simulink model "E_ZH_Z5"  (R2025a)
settings: Solver=VariableStepAuto  StartTime=0.0  StopTime=10.0  RelTol=1e-3
libraries: simulink x2, ZH_Z x1
settings Model: Creator=Szalay  LastModifiedBy=Szalay
settings RTWCC: RTWVerbose=off

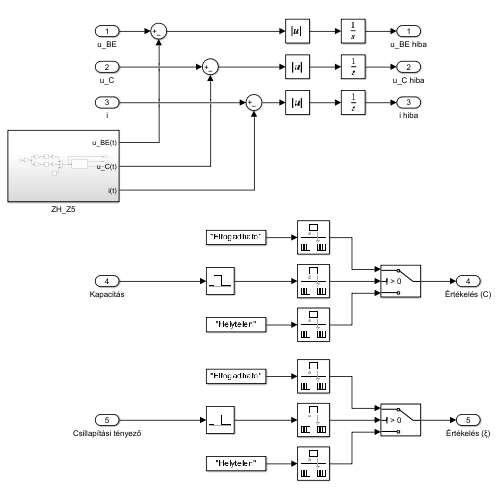
[thumbnail: Simulink's stored preview of the top-level diagram]
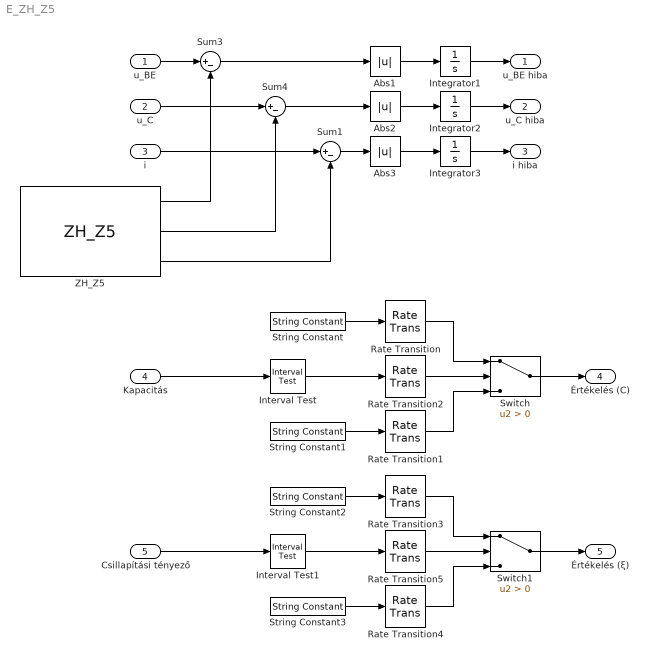
== system E_ZH_Z5 ==
  u_BE : Inport  OutDataTypeStr=double  PortDimensions=1
  u_C : Inport  Port=2  OutDataTypeStr=double  PortDimensions=1
  i : Inport  Port=3  OutDataTypeStr=double  PortDimensions=1
  Kapacitás : Inport  Port=4  OutDataTypeStr=double  PortDimensions=1
  Csillapítási tényező : Inport  Port=5  OutDataTypeStr=double  PortDimensions=1
  Abs1 : Abs  SaturateOnIntegerOverflow=off
  Abs2 : Abs  SaturateOnIntegerOverflow=off
  Abs3 : Abs  SaturateOnIntegerOverflow=off
  Integrator1 : Integrator
  Integrator2 : Integrator
  Integrator3 : Integrator
  Interval Test : simulink/Logic and Bit Operations/Interval Test  IntervalClosedRight=on  uplimit=1.25e-6 * 1.01  IntervalClosedLeft=on  lowlimit=1.25e-6 * 0.99  OutDataTypeStr=boolean
  Interval Test1 : simulink/Logic and Bit Operations/Interval Test  IntervalClosedRight=on  uplimit=0.05 * 1.01  IntervalClosedLeft=on  lowlimit=0.05 * 0.99  OutDataTypeStr=boolean
  Rate Transition{,1..5} (6 alike) : RateTransition  OutPortSampleTime=100e-3
  String Constant : StringConstant  String="\"Elfogadható\""
  String Constant1 : StringConstant  String="\"Helytelen\""
  String Constant2 : StringConstant  String="\"Elfogadható\""
  String Constant3 : StringConstant  String="\"Helytelen\""
  Sum1 : Sum  Inputs=|+-
  Sum3 : Sum  Inputs=|+-
  Sum4 : Sum  Inputs=|+-
  Switch : Switch  Criteria=u2 > Threshold  SaturateOnIntegerOverflow=off  InputSameDT=off
  Switch1 : Switch  Criteria=u2 > Threshold  SaturateOnIntegerOverflow=off  InputSameDT=off
  ZH_Z5 : ZH_Z/ZH_Z5  SystemSampleTime=-1  VariantActivationTime=update diagram  EmptyChoice=off  PassThrough=off  PassThroughVariantControl=(default)  EmptyChoiceVariantControl=(default)  AllowFlexibleInterface=on  Latency=0  AutoFrameSizeCalculation=off
  u_BE hiba : Outport  OutDataTypeStr=double  PortDimensions=1  SampleTime=0
  u_C hiba : Outport  Port=2  OutDataTypeStr=double  PortDimensions=1  SampleTime=0
  i hiba : Outport  Port=3  OutDataTypeStr=double  PortDimensions=1  SampleTime=0
  Értékelés (C) : Outport  Port=4  OutDataTypeStr=string  PortDimensions=1
  Értékelés (ξ) : Outport  Port=5  OutDataTypeStr=string  PortDimensions=1
  wires:
  Integrator1/1 -> u_BE hiba/1
  u_BE/1 -> Sum3/1
  Abs2/1 -> Integrator2/1
  Integrator2/1 -> u_C hiba/1
  Sum3/1 -> Abs1/1
  Sum4/1 -> Abs2/1
  u_C/1 -> Sum4/1
  Abs1/1 -> Integrator1/1
  Integrator3/1 -> i hiba/1
  Abs3/1 -> Integrator3/1
  Sum1/1 -> Abs3/1
  i/1 -> Sum1/1
  ZH_Z5/1 -> Sum3/2
  ZH_Z5/2 -> Sum4/2
  ZH_Z5/3 -> Sum1/2
  Rate Transition2/1 -> Switch/2
  String Constant/1 -> Rate Transition/1
  Kapacitás/1 -> Interval Test/1
  Interval Test/1 -> Rate Transition2/1
  Rate Transition1/1 -> Switch/3
  Switch/1 -> Értékelés (C)/1
  String Constant1/1 -> Rate Transition1/1
  Rate Transition/1 -> Switch/1
  Rate Transition3/1 -> Switch1/1
  String Constant3/1 -> Rate Transition4/1
  Switch1/1 -> Értékelés (ξ)/1
  Rate Transition4/1 -> Switch1/3
  Interval Test1/1 -> Rate Transition5/1
  Csillapítási tényező/1 -> Interval Test1/1
  String Constant2/1 -> Rate Transition3/1
  Rate Transition5/1 -> Switch1/2
